simulink model "AVR_Mu_synthesis__"  (R2022a)
settings: Solver=VariableStepAuto  StartTime=0.0  StopTime=60  RelTol=1e-3
libraries: simulink x1
settings Model: Creator=asus  LastModifiedBy=asus

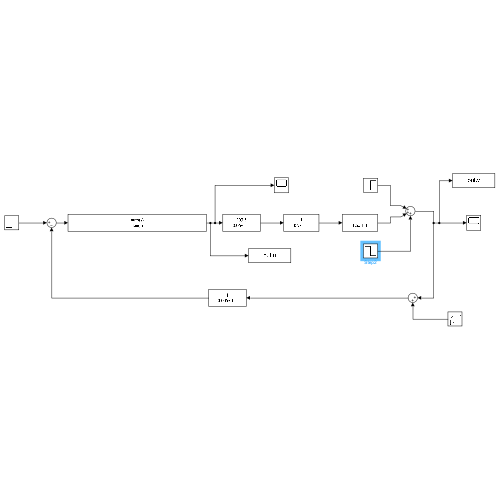
[thumbnail: Simulink's stored preview of the top-level diagram]
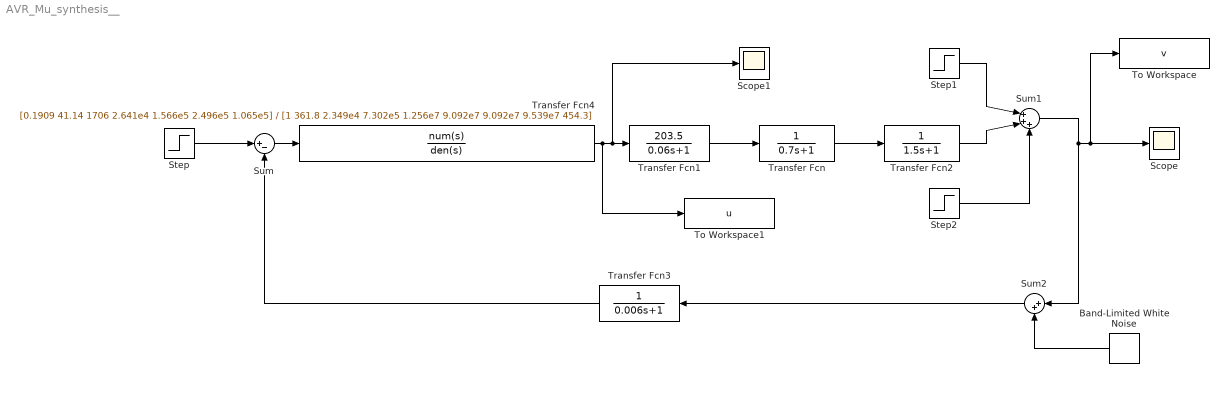
== system AVR_Mu_synthesis__ ==
  Band-Limited White Noise : simulink/Sources/Band-Limited White Noise  Cov=[0]  Ts=0.1  seed=[23341]
  Scope : Scope
  Scope1 : Scope
  Step : Step  Time=0  SampleTime=0
  Step1 : Step  Time=20  SampleTime=0
  Step2 : Step  Time=40  After=-1  SampleTime=0
  Sum : Sum  Inputs=|+-
  Sum1 : Sum  Inputs=|+++
  Sum2 : Sum  Inputs=|++
  To Workspace : ToWorkspace  VariableName=v  SaveFormat=Timeseries  SampleTime=-1
  To Workspace1 : ToWorkspace  VariableName=u  SaveFormat=Timeseries  SampleTime=-1
  Transfer Fcn : TransferFcn  Denominator=[0.7 1]
  Transfer Fcn1 : TransferFcn  Numerator=[203.5]  Denominator=[0.06 1]
  Transfer Fcn2 : TransferFcn  Denominator=[1.5 1]
  Transfer Fcn3 : TransferFcn  Denominator=[0.006 1]
  Transfer Fcn4 : TransferFcn  Numerator=[0.1909 41.14 1706 2.641e4 1.566e5 2.496e5 1.065e5]  Denominator=[1 361.8 2.349e4 7.302e5 1.256e7 9.092e7 9.092e7 9.539e7 454.3]
  wires:
  Band-Limited White Noise/1 -> Sum2/2
  Sum1/1 -> Sum2/1, To Workspace/1, Scope/1
  Step/1 -> Sum/1
  Transfer Fcn2/1 -> Sum1/2
  Step1/1 -> Sum1/1
  Transfer Fcn/1 -> Transfer Fcn2/1
  Transfer Fcn1/1 -> Transfer Fcn/1
  Transfer Fcn3/1 -> Sum/2
  Sum2/1 -> Transfer Fcn3/1
  Sum/1 -> Transfer Fcn4/1
  Step2/1 -> Sum1/3
  Transfer Fcn4/1 -> To Workspace1/1, Scope1/1, Transfer Fcn1/1
